simulink model "real_resource_shared_QR_model"  (R2018b)
settings: Solver=FixedStepDiscrete  StartTime=0.0  StopTime=inf  RelTol=1e-3
InitFcn:
  | % Load some variables if running without a test script
  | if ~exist('A','var') || ~exist('B','var') || ~exist('m','var') || ~exist('n','var') || ~exist('p','var') || ~exist('NumberOfCORDICIterations','var')
  |   m = 4; % Number of rows of A and B.
  |   n = 4; % Number of columns of A.
  |   p = 4; % Number of columns of B.
  |   NumberOfCORDICIterations = 52;
  |   A = 2*rand(m,n)-1;
  |   B = 2*rand(m,p)-1;
  | end
libraries: hdlsllib x9, simulink x2
settings Model: DataTypeOverride=Off  Creator=tbryan  LastModifiedBy=tbryan
settings DataIOCC: LimitDataPoints=on  SaveOutput=off  SaveTime=off
settings OptimizationCC: BlockReduction=off  ConditionallyExecuteInputs=off  DefaultParameterBehavior=Inlined  EnhancedBackFolding=on  StrengthReduction=on  PassReuseOutputArgsAs=Individual arguments  OptimizeBlockOrder=speed  DifferentSizesBufferReuse=on
settings DebuggingCC: AlgebraicLoopMsg=error  SingleTaskRateTransMsg=error  IntegerOverflowMsg=none  ParameterDowncastMsg=none  ParameterOverflowMsg=none  ParameterPrecisionLossMsg=none  ParameterTunabilityLossMsg=error  AllowSymbolicDim=off  LibraryContextMissingDiagnostic=none  StrictBusMsg=ErrorOnBusTreatedAsVector  SFUnexpectedBacktrackingDiag=warning  SFNoUnconditionalDefaultTransitionDiag=warning  SFExecutionAtInitializationDiag=none  IntegerSaturationMsg=none
settings HardwareCC: ProdBitPerPointer=32  ProdBitPerSizeT=32  ProdBitPerPtrDiffT=32  ProdLargestAtomicFloat=None  ProdIntDivRoundTo=Undefined  ProdEndianess=Unspecified  ProdWordSize=32  ProdHWDeviceType=ASIC/FPGA->ASIC/FPGA  TargetBitPerLong=64  TargetBitPerPointer=64  TargetBitPerSizeT=64  TargetBitPerPtrDiffT=64  TargetLongLongMode=on  TargetIntDivRoundTo=Zero  TargetEndianess=LittleEndian  TargetWordSize=64  TargetHWDeviceType=Custom Processor->MATLAB Host Computer  ProdEqTarget=off
settings SFSimCC: SimUseLocalCustomCode=off  MATLABDynamicMemAlloc=off
settings RTWCC: SystemTargetFile=ert.tlc  GenCodeOnly=on  TemplateMakefile=ert_default_tmf  GenerateReport=on  RTWUseLocalCustomCode=off  IncludeHyperlinkInReport=on  LaunchReport=on  GenerateTraceInfo=on  GenerateTraceReport=on  GenerateTraceReportSl=on  GenerateTraceReportSf=on  GenerateTraceReportEml=on
settings CodeAppCC: ForceParamTrailComments=on  IgnoreCustomStorageClasses=off  OperatorAnnotations=on  SimulinkDataObjDesc=on  SFDataObjDesc=on  InsertBlockDesc=on
settings ERTTargetCC: GenerateSampleERTMain=on  InlinedParameterPlacement=NonHierarchical  ERTCustomFileTemplate=example_file_process.tlc
settings ConfigComp: CovScope=ReferencedModels  CovMetricSettings=dw  CovHtmlReporting=on  CovSaveCumulativeToWorkspaceVar=on  CovSaveSingleToWorkspaceVar=on  CovExternalEMLEnable=off  CovSFcnEnable=off

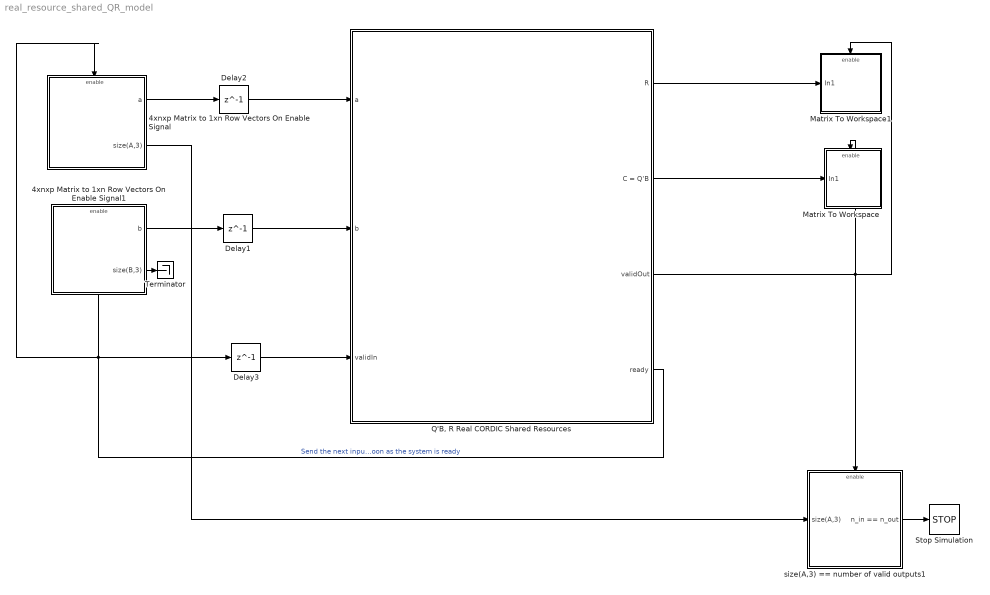
== system real_resource_shared_QR_model ==
  4xnxp Matrix to 1xn Row Vectors On Enable Signal : Subsystem  TreatAsAtomicUnit=on  mask{Matrix=A}
      mask init:
      | obj = get_param(gcbh,'object');
      | constObj = get_param([gcb '/Constant'],'object');
      | constObj.Value = obj.Matrix;
      mask Display: disp(Matrix);
  4xnxp Matrix to 1xn Row Vectors On Enable Signal1 : Subsystem  TreatAsAtomicUnit=on  mask{Matrix=B}
      mask init:
      | obj = get_param(gcbh,'object');
      | constObj = get_param([gcb '/Constant'],'object');
      | constObj.Value = obj.Matrix;
      mask Display: disp(Matrix);
  Delay1 : Delay  DelayLength=1  SampleTime=1
  Delay2 : Delay  DelayLength=1  SampleTime=1
  Delay3 : Delay  DelayLength=1  SampleTime=1
  Matrix To Workspace : Subsystem  mask{VariableName=C}
      mask prompts: VariableName "Variable Name:"
      mask init:
      | obj = get_param(gcbh,'object');
      | twObj = get_param([gcb '/To Workspace'],'object');
      | twObj.VariableName = obj.VariableName;
      mask Display: disp([VariableName,' = Q'' * B']);
  Matrix To Workspace1 : Subsystem  mask{VariableName=R}
      mask prompts: VariableName "Variable Name:"
      mask init:
      | obj = get_param(gcbh,'object');
      | twObj = get_param([gcb '/To Workspace'],'object');
      | twObj.VariableName = obj.VariableName;
      mask Display: disp(VariableName);
  "Q'B, R Real CORDIC Shared Resources" : Subsystem  TreatAsAtomicUnit=on  mask{NumberOfCORDICIterations=NumberOfCORDICIterations, m=m, n=n, p=p}
      mask prompts: NumberOfCORDICIterations "Number of CORDIC Iterations"; m "Number of rows of A and B"; n "Number of columns of A"; p "Number of columns of B"
      mask Display: disp('NumberOfCordicIterations');
  Stop Simulation : Stop
  Terminator : Terminator
  size(A,3) == number of valid outputs1 : Subsystem  TreatAsAtomicUnit=on
  wires:
  4xnxp Matrix to 1xn Row Vectors On Enable Signal/2(size(A,3)) -> size(A,3) == number of valid outputs1/1(size(A,3))
  size(A,3) == number of valid outputs1/1(n_in == n_out) -> Stop Simulation/1
  "Q'B, R Real CORDIC Shared Resources"/2(C = Q'B) -> Matrix To Workspace/1(In1)
  "Q'B, R Real CORDIC Shared Resources"/3(validOut) -> Matrix To Workspace1/Enable, Matrix To Workspace/Enable, size(A,3) == number of valid outputs1/Enable
  4xnxp Matrix to 1xn Row Vectors On Enable Signal/1(a) -> Delay2/1
  4xnxp Matrix to 1xn Row Vectors On Enable Signal1/1(b) -> Delay1/1
  Delay1/1 -> "Q'B, R Real CORDIC Shared Resources"/2(b)
  Delay2/1 -> "Q'B, R Real CORDIC Shared Resources"/1(a)
  Delay3/1 -> "Q'B, R Real CORDIC Shared Resources"/3(validIn)
  "Q'B, R Real CORDIC Shared Resources"/1(R) -> Matrix To Workspace1/1(In1)
  4xnxp Matrix to 1xn Row Vectors On Enable Signal1/2(size(B,3)) -> Terminator/1
  "Q'B, R Real CORDIC Shared Resources"/4(ready) -> 4xnxp Matrix to 1xn Row Vectors On Enable Signal/Enable, 4xnxp Matrix to 1xn Row Vectors On Enable Signal1/Enable, Delay3/1  "Send the next input in as soon as the system is ready"

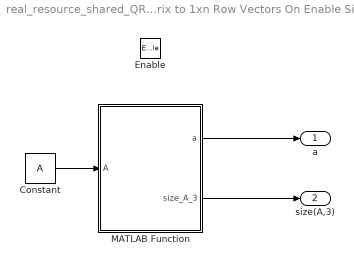
== system real_resource_shared_QR_model/4xnxp Matrix to 1xn Row Vectors On Enable Signal ==
  Enable : EnablePort
  Constant : Constant  Value=A
  MATLAB Function : MATLAB Function  TreatAsAtomicUnit=on
  a : Outport
  size(A,3) : Outport  Port=2
  wires:
  MATLAB Function/1(a) -> a/1
  Constant/1 -> MATLAB Function/1(A)
  MATLAB Function/2(size_A_3) -> size(A,3)/1

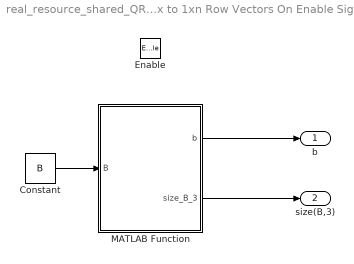
== system real_resource_shared_QR_model/4xnxp Matrix to 1xn Row Vectors On Enable Signal1 ==
  Enable : EnablePort
  Constant : Constant  Value=B
  MATLAB Function : MATLAB Function  TreatAsAtomicUnit=on
  b : Outport
  size(B,3) : Outport  Port=2
  wires:
  MATLAB Function/1(b) -> b/1
  Constant/1 -> MATLAB Function/1(B)
  MATLAB Function/2(size_B_3) -> size(B,3)/1

== system real_resource_shared_QR_model/Matrix To Workspace ==
  In1 : Inport
  Enable : EnablePort
  To Workspace : ToWorkspace  VariableName=C  SampleTime=-1
  wires:
  In1/1 -> To Workspace/1

== system real_resource_shared_QR_model/Matrix To Workspace1 ==
  In1 : Inport
  Enable : EnablePort
  To Workspace : ToWorkspace  VariableName=R  SampleTime=-1
  wires:
  In1/1 -> To Workspace/1

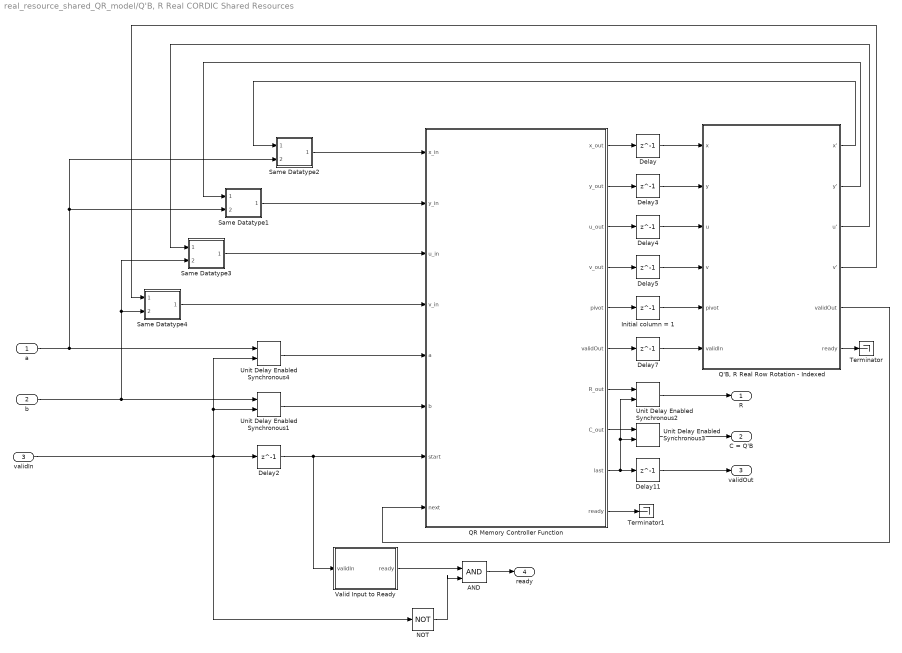
== system real_resource_shared_QR_model/Q'B, R Real CORDIC Shared Resources ==
  a : Inport
  b : Inport  Port=2
  validIn : Inport  Port=3
  AND : Logic  IconShape=distinctive  AllPortsSameDT=off  OutDataTypeStr=boolean
  Delay{,2..5} (5 alike) : Delay  DelayLength=1
  Delay11 : Delay  DelayLength=1  InitialCondition=0
  Delay7 : Delay  DelayLength=1  InitialCondition=0
  Initial column = 1 : Delay  DelayLength=1  InitialCondition=1
  NOT : Logic  Operator=NOT  IconShape=distinctive  AllPortsSameDT=off  OutDataTypeStr=boolean
  "Q'B, R Real Row Rotation - Indexed" : Subsystem  TreatAsAtomicUnit=on  mask{NumberOfCORDICIterations=NumberOfCORDICIterations}
      mask prompts: NumberOfCORDICIterations "Number of CORDIC Iterations"
  QR Memory Controller Function : MATLAB Function  TreatAsAtomicUnit=on
  Same Datatype1 : Subsystem  TreatAsAtomicUnit=on
  Same Datatype2 : Subsystem  TreatAsAtomicUnit=on
  Same Datatype3 : Subsystem  TreatAsAtomicUnit=on
  Same Datatype4 : Subsystem  TreatAsAtomicUnit=on
  Terminator : Terminator
  Terminator1 : Terminator
  Unit Delay Enabled Synchronous{1..4} (4 alike) : hdlsllib/Discrete/Unit Delay Enabled Synchronous  InitialCondition=0.0  SampleTime=-1
      settings: SourceProductName=HDL Coder  SourceProductBaseCode=HD
  Valid Input to Ready : Subsystem  TreatAsAtomicUnit=on  mask{NumberOfCORDICIterations=NumberOfCORDICIterations, m=m, n=n}
      mask prompts: NumberOfCORDICIterations "Number of CORDIC Iterations"; m "Number of rows of A"; n "Number of columns of A"
  R : Outport
  C = Q'B : Outport  Port=2
  validOut : Outport  Port=3
  ready : Outport  Port=4
  wires:
  a/1 -> Unit Delay Enabled Synchronous4/1, Same Datatype2/2(Reference), Same Datatype1/2(Reference)
  b/1 -> Unit Delay Enabled Synchronous1/1, Same Datatype3/2(Reference), Same Datatype4/2(Reference)
  Delay2/1 -> Valid Input to Ready/1(validIn), QR Memory Controller Function/7(start)
  "Q'B, R Real Row Rotation - Indexed"/1(x') -> Same Datatype2/1(Data)
  "Q'B, R Real Row Rotation - Indexed"/2(y') -> Same Datatype1/1(Data)
  "Q'B, R Real Row Rotation - Indexed"/3(u') -> Same Datatype3/1(Data)
  "Q'B, R Real Row Rotation - Indexed"/4(v') -> Same Datatype4/1(Data)
  validIn/1 -> NOT/1, Unit Delay Enabled Synchronous1/2, Unit Delay Enabled Synchronous4/2, Delay2/1
  Same Datatype2/1(DataOut) -> QR Memory Controller Function/1(x_in)
  Same Datatype1/1(DataOut) -> QR Memory Controller Function/2(y_in)
  Same Datatype3/1(DataOut) -> QR Memory Controller Function/3(u_in)
  Same Datatype4/1(DataOut) -> QR Memory Controller Function/4(v_in)
  Unit Delay Enabled Synchronous4/1 -> QR Memory Controller Function/5(a)
  "Q'B, R Real Row Rotation - Indexed"/6(ready) -> Terminator/1
  "Q'B, R Real Row Rotation - Indexed"/5(validOut) -> QR Memory Controller Function/8(next)
  QR Memory Controller Function/1(x_out) -> Delay/1
  QR Memory Controller Function/2(y_out) -> Delay3/1
  QR Memory Controller Function/3(u_out) -> Delay4/1
  QR Memory Controller Function/4(v_out) -> Delay5/1
  QR Memory Controller Function/5(pivot) -> Initial column = 1/1
  QR Memory Controller Function/6(validOut) -> Delay7/1
  Delay/1 -> "Q'B, R Real Row Rotation - Indexed"/1(x)
  Delay3/1 -> "Q'B, R Real Row Rotation - Indexed"/2(y)
  Delay4/1 -> "Q'B, R Real Row Rotation - Indexed"/3(u)
  Delay5/1 -> "Q'B, R Real Row Rotation - Indexed"/4(v)
  Initial column = 1/1 -> "Q'B, R Real Row Rotation - Indexed"/5(pivot)
  Delay7/1 -> "Q'B, R Real Row Rotation - Indexed"/6(validIn)
  QR Memory Controller Function/7(R_out) -> Unit Delay Enabled Synchronous2/1
  QR Memory Controller Function/8(C_out) -> Unit Delay Enabled Synchronous3/1
  QR Memory Controller Function/9(last) -> Unit Delay Enabled Synchronous3/2, Unit Delay Enabled Synchronous2/2, Delay11/1
  Delay11/1 -> validOut/1
  Unit Delay Enabled Synchronous1/1 -> QR Memory Controller Function/6(b)
  Unit Delay Enabled Synchronous2/1 -> R/1
  Unit Delay Enabled Synchronous3/1 -> C = Q'B/1
  QR Memory Controller Function/10(ready) -> Terminator1/1
  AND/1 -> ready/1
  Valid Input to Ready/1(ready) -> AND/1
  NOT/1 -> AND/2

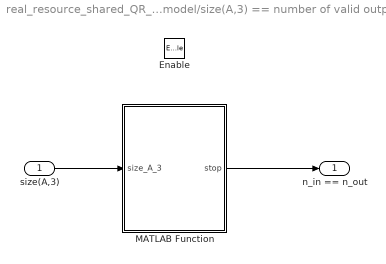
== system real_resource_shared_QR_model/size(A,3) == number of valid outputs1 ==
  size(A,3) : Inport
  Enable : EnablePort
  MATLAB Function : MATLAB Function  TreatAsAtomicUnit=on
  n_in == n_out : Outport
  wires:
  MATLAB Function/1(stop) -> n_in == n_out/1
  size(A,3)/1 -> MATLAB Function/1(size_A_3)

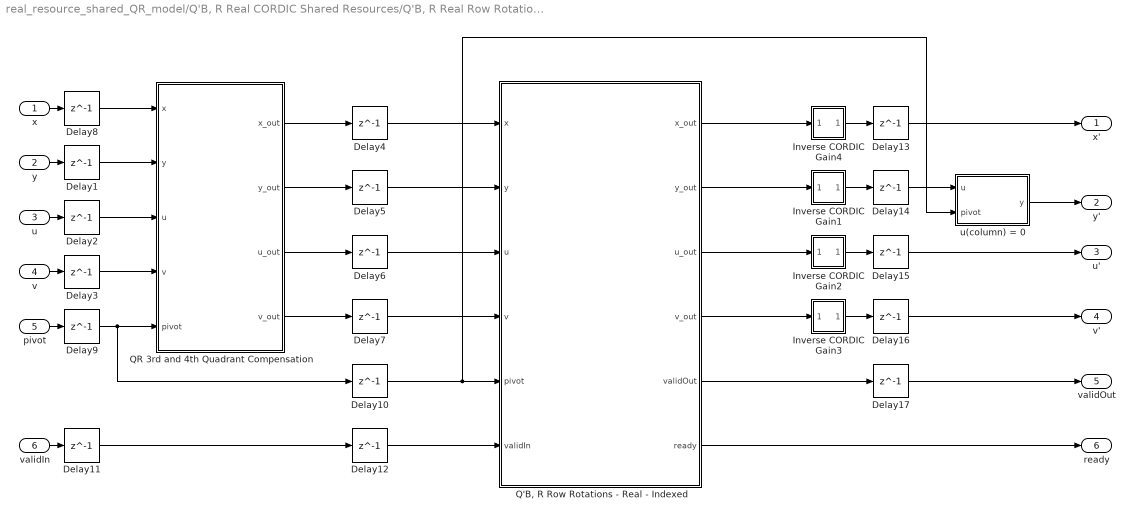
== system real_resource_shared_QR_model/Q'B, R Real CORDIC Shared Resources/Q'B, R Real Row Rotation - Indexed ==
  x : Inport
  y : Inport  Port=2
  u : Inport  Port=3
  v : Inport  Port=4
  pivot : Inport  Port=5
  validIn : Inport  Port=6
  Delay{1..8,11..17} (15 alike) : Delay  DelayLength=1
  Delay10 : Delay  DelayLength=1  InitialCondition=1
  Delay9 : Delay  DelayLength=1  InitialCondition=1
  Inverse CORDIC Gain1 : Subsystem  TreatAsAtomicUnit=on  mask{NumberOfCORDICIterations=NumberOfCORDICIterations}
      mask prompts: NumberOfCORDICIterations "Number of CORDIC Iterations"
      mask Display: disp('1/An')
  Inverse CORDIC Gain2 : Subsystem  TreatAsAtomicUnit=on  mask{NumberOfCORDICIterations=NumberOfCORDICIterations}
      mask prompts: NumberOfCORDICIterations "Number of CORDIC Iterations"
      mask Display: disp('1/An')
  Inverse CORDIC Gain3 : Subsystem  TreatAsAtomicUnit=on  mask{NumberOfCORDICIterations=NumberOfCORDICIterations}
      mask prompts: NumberOfCORDICIterations "Number of CORDIC Iterations"
      mask Display: disp('1/An')
  Inverse CORDIC Gain4 : Subsystem  TreatAsAtomicUnit=on  mask{NumberOfCORDICIterations=NumberOfCORDICIterations}
      mask prompts: NumberOfCORDICIterations "Number of CORDIC Iterations"
      mask Display: disp('1/An')
  "Q'B, R Row Rotations - Real - Indexed" : Subsystem  TreatAsAtomicUnit=on  mask{NumberOfCORDICIterations=NumberOfCORDICIterations}
      mask prompts: NumberOfCORDICIterations "Number of CORDIC Iterations"
  QR 3rd and 4th Quadrant Compensation : MATLAB Function  TreatAsAtomicUnit=on
  u(column) = 0 : MATLAB Function  TreatAsAtomicUnit=on
  x' : Outport
  y' : Outport  Port=2
  u' : Outport  Port=3
  v' : Outport  Port=4
  validOut : Outport  Port=5
  ready : Outport  Port=6
  wires:
  u(column) = 0/1(y) -> y'/1
  Delay9/1 -> Delay10/1, QR 3rd and 4th Quadrant Compensation/5(pivot)
  pivot/1 -> Delay9/1
  Delay10/1 -> u(column) = 0/2(pivot), "Q'B, R Row Rotations - Real - Indexed"/5(pivot)
  Delay12/1 -> "Q'B, R Row Rotations - Real - Indexed"/6(validIn)
  Delay3/1 -> QR 3rd and 4th Quadrant Compensation/4(v)
  Delay1/1 -> QR 3rd and 4th Quadrant Compensation/2(y)
  y/1 -> Delay1/1
  Delay2/1 -> QR 3rd and 4th Quadrant Compensation/3(u)
  Delay8/1 -> QR 3rd and 4th Quadrant Compensation/1(x)
  "Q'B, R Row Rotations - Real - Indexed"/6(ready) -> ready/1
  Delay17/1 -> validOut/1
  "Q'B, R Row Rotations - Real - Indexed"/5(validOut) -> Delay17/1
  Delay16/1 -> v'/1
  Delay15/1 -> u'/1
  Delay13/1 -> x'/1
  Delay11/1 -> Delay12/1
  validIn/1 -> Delay11/1
  "Q'B, R Row Rotations - Real - Indexed"/2(y_out) -> Inverse CORDIC Gain1/1(In1)
  Delay14/1 -> u(column) = 0/1(u)
  Inverse CORDIC Gain1/1(Out1) -> Delay14/1
  "Q'B, R Row Rotations - Real - Indexed"/4(v_out) -> Inverse CORDIC Gain3/1(In1)
  "Q'B, R Row Rotations - Real - Indexed"/3(u_out) -> Inverse CORDIC Gain2/1(In1)
  "Q'B, R Row Rotations - Real - Indexed"/1(x_out) -> Inverse CORDIC Gain4/1(In1)
  Delay7/1 -> "Q'B, R Row Rotations - Real - Indexed"/4(v)
  Delay6/1 -> "Q'B, R Row Rotations - Real - Indexed"/3(u)
  Delay5/1 -> "Q'B, R Row Rotations - Real - Indexed"/2(y)
  Delay4/1 -> "Q'B, R Row Rotations - Real - Indexed"/1(x)
  Inverse CORDIC Gain2/1(Out1) -> Delay15/1
  v/1 -> Delay3/1
  u/1 -> Delay2/1
  x/1 -> Delay8/1
  Inverse CORDIC Gain4/1(Out1) -> Delay13/1
  Inverse CORDIC Gain3/1(Out1) -> Delay16/1
  QR 3rd and 4th Quadrant Compensation/4(v_out) -> Delay7/1
  QR 3rd and 4th Quadrant Compensation/2(y_out) -> Delay5/1
  QR 3rd and 4th Quadrant Compensation/3(u_out) -> Delay6/1
  QR 3rd and 4th Quadrant Compensation/1(x_out) -> Delay4/1

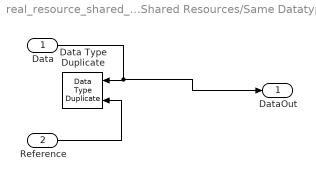
== system real_resource_shared_QR_model/Q'B, R Real CORDIC Shared Resources/Same Datatype1 ==
  Data : Inport
  Reference : Inport  Port=2
  Data Type Duplicate : DataTypeDuplicate
  DataOut : Outport
  wires:
  Data/1 -> Data Type Duplicate/1, DataOut/1
  Reference/1 -> Data Type Duplicate/2

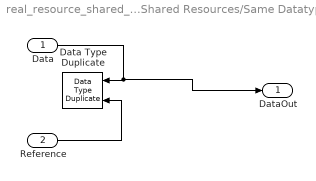
== system real_resource_shared_QR_model/Q'B, R Real CORDIC Shared Resources/Same Datatype2 ==
  Data : Inport
  Reference : Inport  Port=2
  Data Type Duplicate : DataTypeDuplicate
  DataOut : Outport
  wires:
  Data/1 -> Data Type Duplicate/1, DataOut/1
  Reference/1 -> Data Type Duplicate/2

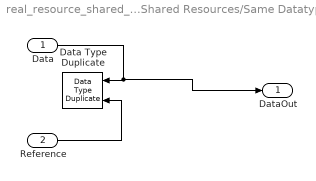
== system real_resource_shared_QR_model/Q'B, R Real CORDIC Shared Resources/Same Datatype3 ==
  Data : Inport
  Reference : Inport  Port=2
  Data Type Duplicate : DataTypeDuplicate
  DataOut : Outport
  wires:
  Data/1 -> Data Type Duplicate/1, DataOut/1
  Reference/1 -> Data Type Duplicate/2

== system real_resource_shared_QR_model/Q'B, R Real CORDIC Shared Resources/Same Datatype4 ==
  Data : Inport
  Reference : Inport  Port=2
  Data Type Duplicate : DataTypeDuplicate
  DataOut : Outport
  wires:
  Data/1 -> Data Type Duplicate/1, DataOut/1
  Reference/1 -> Data Type Duplicate/2

== system real_resource_shared_QR_model/Q'B, R Real CORDIC Shared Resources/Valid Input to Ready ==
  validIn : Inport
  MATLAB Function : MATLAB Function  TreatAsAtomicUnit=on
  ready : Outport
  wires:
  validIn/1 -> MATLAB Function/1(validIn)
  MATLAB Function/1(ready) -> ready/1

== system real_resource_shared_QR_model/Q'B, R Real CORDIC Shared Resources/Q'B, R Real Row Rotation - Indexed/Inverse CORDIC Gain1 ==
  In1 : Inport
  Inverse CORDIC Gain : Gain  Gain=1/prod(sqrt(1+2.^(-2*(0:double(NumberOfCORDICIterations)-1))))  OutDataTypeStr=Inherit: Same as input
  Out1 : Outport
  wires:
  Inverse CORDIC Gain/1 -> Out1/1
  In1/1 -> Inverse CORDIC Gain/1

== system real_resource_shared_QR_model/Q'B, R Real CORDIC Shared Resources/Q'B, R Real Row Rotation - Indexed/Inverse CORDIC Gain2 ==
  In1 : Inport
  Inverse CORDIC Gain : Gain  Gain=1/prod(sqrt(1+2.^(-2*(0:double(NumberOfCORDICIterations)-1))))  OutDataTypeStr=Inherit: Same as input
  Out1 : Outport
  wires:
  Inverse CORDIC Gain/1 -> Out1/1
  In1/1 -> Inverse CORDIC Gain/1

== system real_resource_shared_QR_model/Q'B, R Real CORDIC Shared Resources/Q'B, R Real Row Rotation - Indexed/Inverse CORDIC Gain3 ==
  In1 : Inport
  Inverse CORDIC Gain : Gain  Gain=1/prod(sqrt(1+2.^(-2*(0:double(NumberOfCORDICIterations)-1))))  OutDataTypeStr=Inherit: Same as input
  Out1 : Outport
  wires:
  Inverse CORDIC Gain/1 -> Out1/1
  In1/1 -> Inverse CORDIC Gain/1

== system real_resource_shared_QR_model/Q'B, R Real CORDIC Shared Resources/Q'B, R Real Row Rotation - Indexed/Inverse CORDIC Gain4 ==
  In1 : Inport
  Inverse CORDIC Gain : Gain  Gain=1/prod(sqrt(1+2.^(-2*(0:double(NumberOfCORDICIterations)-1))))  OutDataTypeStr=Inherit: Same as input
  Out1 : Outport
  wires:
  Inverse CORDIC Gain/1 -> Out1/1
  In1/1 -> Inverse CORDIC Gain/1

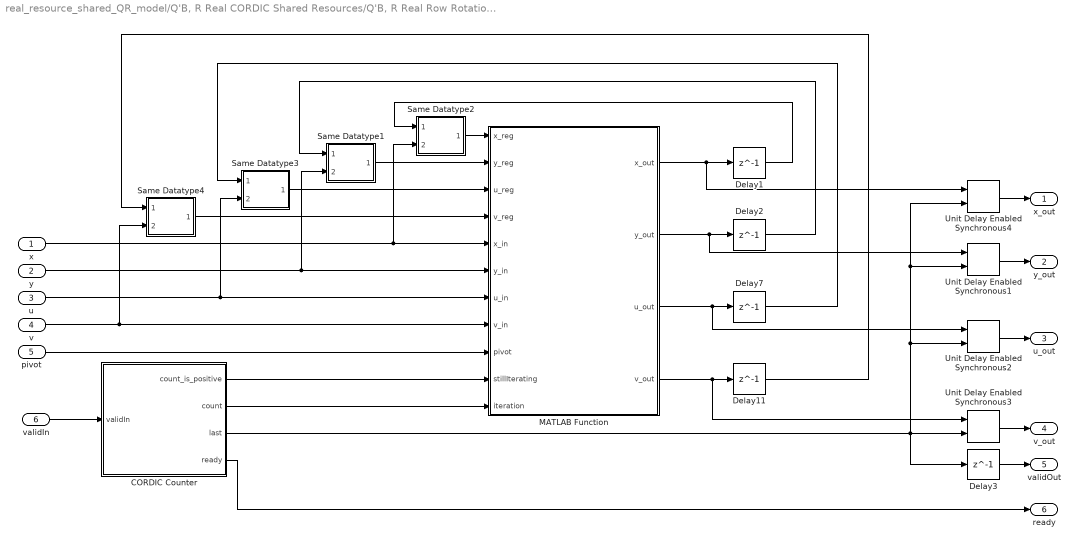
== system real_resource_shared_QR_model/Q'B, R Real CORDIC Shared Resources/Q'B, R Real Row Rotation - Indexed/Q'B, R Row Rotations - Real - Indexed ==
  x : Inport
  y : Inport  Port=2
  u : Inport  Port=3
  v : Inport  Port=4
  pivot : Inport  Port=5
  validIn : Inport  Port=6
  CORDIC Counter : Subsystem  mask{NumberOfCORDICIterations=NumberOfCORDICIterations}
      mask prompts: NumberOfCORDICIterations "Number of CORDIC Iterations"
  Delay{1..3,7,11} (5 alike) : Delay  DelayLength=1
  MATLAB Function : MATLAB Function  TreatAsAtomicUnit=on
  Same Datatype1 : Subsystem  TreatAsAtomicUnit=on
  Same Datatype2 : Subsystem  TreatAsAtomicUnit=on
  Same Datatype3 : Subsystem  TreatAsAtomicUnit=on
  Same Datatype4 : Subsystem  TreatAsAtomicUnit=on
  Unit Delay Enabled Synchronous{1..4} (4 alike) : hdlsllib/Discrete/Unit Delay Enabled Synchronous  InitialCondition=0.0  SampleTime=-1
      settings: SourceProductName=HDL Coder  SourceProductBaseCode=HD
  x_out : Outport
  y_out : Outport  Port=2
  u_out : Outport  Port=3
  v_out : Outport  Port=4
  validOut : Outport  Port=5
  ready : Outport  Port=6
  wires:
  pivot/1 -> MATLAB Function/9(pivot)
  Unit Delay Enabled Synchronous4/1 -> x_out/1
  Unit Delay Enabled Synchronous1/1 -> y_out/1
  Unit Delay Enabled Synchronous2/1 -> u_out/1
  Unit Delay Enabled Synchronous3/1 -> v_out/1
  validIn/1 -> CORDIC Counter/1(validIn)
  CORDIC Counter/4(ready) -> ready/1
  CORDIC Counter/3(last) -> Unit Delay Enabled Synchronous2/2, Unit Delay Enabled Synchronous4/2, Unit Delay Enabled Synchronous1/2, Unit Delay Enabled Synchronous3/2, Delay3/1
  Delay3/1 -> validOut/1
  Same Datatype4/1(DataOut) -> MATLAB Function/4(v_reg)
  Same Datatype3/1(DataOut) -> MATLAB Function/3(u_reg)
  Same Datatype1/1(DataOut) -> MATLAB Function/2(y_reg)
  v/1 -> MATLAB Function/8(v_in), Same Datatype4/2(Reference)
  u/1 -> MATLAB Function/7(u_in), Same Datatype3/2(Reference)
  y/1 -> MATLAB Function/6(y_in), Same Datatype1/2(Reference)
  x/1 -> MATLAB Function/5(x_in), Same Datatype2/2(Reference)
  Same Datatype2/1(DataOut) -> MATLAB Function/1(x_reg)
  MATLAB Function/4(v_out) -> Unit Delay Enabled Synchronous3/1, Delay11/1
  MATLAB Function/3(u_out) -> Unit Delay Enabled Synchronous2/1, Delay7/1
  MATLAB Function/2(y_out) -> Unit Delay Enabled Synchronous1/1, Delay2/1
  MATLAB Function/1(x_out) -> Delay1/1, Unit Delay Enabled Synchronous4/1
  CORDIC Counter/2(count) -> MATLAB Function/11(iteration)
  CORDIC Counter/1(count_is_positive) -> MATLAB Function/10(stillIterating)
  Delay11/1 -> Same Datatype4/1(Data)
  Delay7/1 -> Same Datatype3/1(Data)
  Delay2/1 -> Same Datatype1/1(Data)
  Delay1/1 -> Same Datatype2/1(Data)

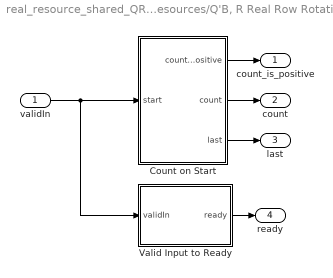
== system real_resource_shared_QR_model/Q'B, R Real CORDIC Shared Resources/Q'B, R Real Row Rotation - Indexed/Q'B, R Row Rotations - Real - Indexed/CORDIC Counter ==
  validIn : Inport
  Count on Start : Subsystem  TreatAsAtomicUnit=on  mask{cmax=NumberOfCORDICIterations - 1}
      mask prompts: cmax "Count Max"
  Valid Input to Ready : Subsystem  TreatAsAtomicUnit=on  mask{NumberOfCORDICIterations=NumberOfCORDICIterations}
      mask prompts: NumberOfCORDICIterations "Number of CORDIC Iterations"
  count_is_positive : Outport
  count : Outport  Port=2
  last : Outport  Port=3
  ready : Outport  Port=4
  wires:
  Valid Input to Ready/1(ready) -> ready/1
  validIn/1 -> Count on Start/1(start), Valid Input to Ready/1(validIn)
  Count on Start/1(count_is_positive) -> count_is_positive/1
  Count on Start/3(last) -> last/1
  Count on Start/2(count) -> count/1

== system real_resource_shared_QR_model/Q'B, R Real CORDIC Shared Resources/Q'B, R Real Row Rotation - Indexed/Q'B, R Row Rotations - Real - Indexed/Same Datatype1 ==
  Data : Inport
  Reference : Inport  Port=2
  Data Type Duplicate : DataTypeDuplicate
  DataOut : Outport
  wires:
  Data/1 -> Data Type Duplicate/1, DataOut/1
  Reference/1 -> Data Type Duplicate/2

== system real_resource_shared_QR_model/Q'B, R Real CORDIC Shared Resources/Q'B, R Real Row Rotation - Indexed/Q'B, R Row Rotations - Real - Indexed/Same Datatype2 ==
  Data : Inport
  Reference : Inport  Port=2
  Data Type Duplicate : DataTypeDuplicate
  DataOut : Outport
  wires:
  Data/1 -> Data Type Duplicate/1, DataOut/1
  Reference/1 -> Data Type Duplicate/2

== system real_resource_shared_QR_model/Q'B, R Real CORDIC Shared Resources/Q'B, R Real Row Rotation - Indexed/Q'B, R Row Rotations - Real - Indexed/Same Datatype3 ==
  Data : Inport
  Reference : Inport  Port=2
  Data Type Duplicate : DataTypeDuplicate
  DataOut : Outport
  wires:
  Data/1 -> Data Type Duplicate/1, DataOut/1
  Reference/1 -> Data Type Duplicate/2

== system real_resource_shared_QR_model/Q'B, R Real CORDIC Shared Resources/Q'B, R Real Row Rotation - Indexed/Q'B, R Row Rotations - Real - Indexed/Same Datatype4 ==
  Data : Inport
  Reference : Inport  Port=2
  Data Type Duplicate : DataTypeDuplicate
  DataOut : Outport
  wires:
  Data/1 -> Data Type Duplicate/1, DataOut/1
  Reference/1 -> Data Type Duplicate/2

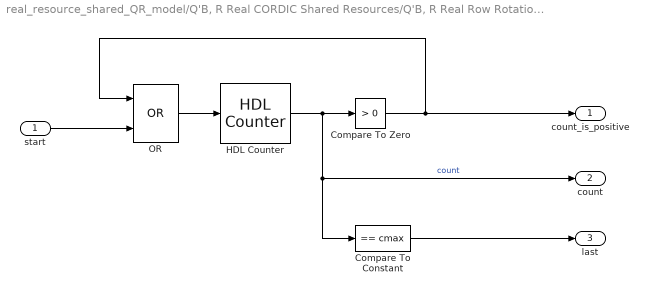
== system real_resource_shared_QR_model/Q'B, R Real CORDIC Shared Resources/Q'B, R Real Row Rotation - Indexed/Q'B, R Row Rotations - Real - Indexed/CORDIC Counter/Count on Start ==
  start : Inport
  Compare To Constant : simulink/Logic and Bit Operations/Compare To Constant  relop===  const=cmax  OutDataTypeStr=boolean
  Compare To Zero : simulink/Logic and Bit Operations/Compare To Zero  relop=>  OutDataTypeStr=boolean
  HDL Counter : hdlsllib/Sources/HDL Counter  CountType=Count limited  CountInit=0  CountStep=1  CountMax=cmax  CountFromType=Initial value  CountFrom=0  CountResetPort=off  CountLoadPort=off  CountEnbPort=on  CountDirPort=off  CountDataType=Unsigned  CountWordLen=nextpow2(cmax+1)  CountFracLen=0  CountSampTime=1
      settings: SourceProductBaseCode=HD
  OR : Logic  Operator=OR  IconShape=distinctive  AllPortsSameDT=off  OutDataTypeStr=boolean
  count_is_positive : Outport
  count : Outport  Port=2
  last : Outport  Port=3
  wires:
  OR/1 -> HDL Counter/1
  Compare To Zero/1 -> OR/1, count_is_positive/1
  start/1 -> OR/2
  HDL Counter/1 -> Compare To Constant/1, count/1, Compare To Zero/1  "count"
  Compare To Constant/1 -> last/1

== system real_resource_shared_QR_model/Q'B, R Real CORDIC Shared Resources/Q'B, R Real Row Rotation - Indexed/Q'B, R Row Rotations - Real - Indexed/CORDIC Counter/Valid Input to Ready ==
  validIn : Inport
  MATLAB Function : MATLAB Function  TreatAsAtomicUnit=on
  ready : Outport
  wires:
  MATLAB Function/1(ready_out) -> ready/1
  validIn/1 -> MATLAB Function/1(validIn)

== matlab function real_resource_shared_QR_model/4xnxp Matrix to 1xn Row Vectors On Enable Signal1/MATLAB Function ==
  settings: fimath=fimath('RoundingMethod','Floor','OverflowAction','Wrap')
  data: b output; B input; size_B_3 output
function [b,size_B_3] = matrix_to_row_vectors_4x4(B)
    persistent p
    if isempty(p)
        p = 1;
    end
    b = reshape(B(:,:,p),1,size(B,1)*size(B,2));
    p = p + 1;
    if p>size(B,3)
        p = 1;
    end
    size_B_3 = size(B,3);
end

== matlab function real_resource_shared_QR_model/Q'B, R Real CORDIC Shared Resources/Q'B, R Real Row Rotation - Indexed/Q'B, R Row Rotations - Real - Indexed/MATLAB Function ==
  settings: fimath=fimath('RoundingMethod','Floor','OverflowAction','Wrap')
  data: x_reg input; y_reg input; u_reg input; v_reg input; x_in input; y_in input; u_in input; x_out output; y_out output; u_out output; v_in input; pivot input size=1; stillIterating input; iteration input size=1; v_out output
function [x_out,y_out,u_out,v_out] = cordic_qr_row_rotation(...
        x_reg,y_reg,u_reg,v_reg,...
        x_in,y_in,u_in,v_in,...
        pivot,...
        stillIterating, iteration)
    % This is one CORDIC rotation for the QR decomposition.
    % In the matrix equation A*X = B
    % x and y form R from A
    % u and v form Q'*B from B
    
    % Initialize output variables
    x_out = x_in;
    y_out = y_in;
    u_out = u_in;
    v_out = v_in;
    
    if pivot <= length(y_in)
        if stillIterating
            % The next values are the previous values from the register
            x = x_reg;
            y = y_reg;
            u = u_reg;
            v = v_reg;
        else
            % The next values are the new input values
            x = x_in;
            y = y_in;
            u = u_in;
            v = v_in;
        end
        
        % Right shift the inputs for CORDIC rotations.
        x1 = bitsra(x, iteration);
        y1 = bitsra(y, iteration);
        u1 = bitsra(u, iteration);
        v1 = bitsra(v, iteration);
        if real(y(pivot)) < 0
            % Counter-clockwise rotation
            x_out(:) = x - y1;
            y_out(:) = y + x1;
            
            u_out(:) = u - v1;
            v_out(:) = v + u1;
        else
            % Clockwise rotation
            x_out(:) = x + y1;
            y_out(:) = y - x1;
            
            u_out(:) = u + v1;
            v_out(:) = v - u1;
        end
    end
end

== matlab function real_resource_shared_QR_model/Q'B, R Real CORDIC Shared Resources/Valid Input to Ready/MATLAB Function ==
  settings: fimath=fimath('RoundingMethod','Floor','OverflowAction','Wrap')
  data: validIn input boolean size=1; ready output boolean size=1; NumberOfCORDICIterations parameter size=1; m parameter size=1; n parameter size=1
function ready = valid_in_ready_out(validIn, NumberOfCORDICIterations,m, n)
    persistent count
    if isempty(count)
        count = uint32(0);
    end
    % Constants
    if m<n
        number_of_lower_triangular_entries = m*(m-1)/2;
    else
        number_of_lower_triangular_entries = n*(n-1)/2 + (m-n)*n;
    end
    count_to_ready = (number_of_lower_triangular_entries+5) * NumberOfCORDICIterations;
    if validIn
        count(:) = 1;
        ready = false;
    elseif count > count_to_ready
        ready = true;
        count(:) = 0;
    elseif count > 0
        count(:) = count + 1;
        ready = false;
    else
        ready = true;
    end
end

== matlab function real_resource_shared_QR_model/Q'B, R Real CORDIC Shared Resources/QR Memory Controller Function ==
  data: x_in input size=[1,n]; y_in input size=[1,n]; u_in input size=[1,p]; v_in input size=[1,p]; a input size=[1,m*n]; x_out output size=[1,n]; b input size=[1,m*p]; start input boolean size=1; next input boolean size=1; y_out output size=[1,n]; u_out output size=[1,p]; v_out output size=[1,p]; pivot output size=1; validOut output; R_out output size=[m,n]; C_out output size=[m,p]; last output boolean size=1; m parameter size=1; n parameter size=1; p parameter size=1; ready output boolean size=1
function [x_out,...
        y_out,...
        u_out,...
        v_out,...
        pivot,...
        validOut,...
        R_out,...
        C_out,...
        last,...
        ready]...
          = qr_memory_controller(...
        x_in,...
        y_in,...
        u_in,...
        v_in,...
        a,...
        b,...
        start,...
        next,...
        m,...
        n,...
        p)
    
    persistent R C i pPivot count pReady
    if isempty(R)
        % Initialize persistent variables
        R = zeros(m,n,'like',a);
        C = zeros(m,p,'like',b);
        pPivot = uint16(1);
        i = uint16(1);
        count = uint16(0);
        pReady = true;
    end
    mn = min(m,n);
    if m<n
        number_of_lower_triangular_entries = m*(m-1)/2;
    else
        number_of_lower_triangular_entries = n*(n-1)/2 + (m-n)*n;
    end
    last = false;
    validOut = false;
    x_out = zeros(1,n,'like',a);
    y_out = zeros(1,n,'like',a);
    u_out = zeros(1,p,'like',b);
    v_out = zeros(1,p,'like',b);
    if start
        count(:) = 1;
        % Start with a new matrix
        % Overwrite A with R
        R(:) = a;
        % Overwrite B with C = Q'B
        C(:) = b;
        % Initial indices
        pPivot(:) = 1;
        i(:) = 2;
        if pPivot<=mn && i<=m
            % Initial rows to operate over
            x_out = R(pPivot,:);
            y_out = R(i,:);
            u_out = C(pPivot,:);
            v_out = C(i,:);
        end
        pReady = false;
        validOut = true;
    elseif next && count ~= 0
        count(:) = count + 1;
        % Update previous pair of rows and get next pair
        if pPivot<=mn && i<=m
            % Update R with previous values
            R(pPivot,:) = x_in;
            R(i,:) = y_in;
            % Update C with previous values
            C(pPivot,:) = u_in;
            C(i,:) = v_in;
            % Increment loop
            i(:) = i + 1;  % Inner loop
            if i > m
                pPivot(:) = pPivot + 1;  % Outer loop
                i(:) = pPivot + 1;
            end
            if pPivot <= mn && i <= m
                % Next rows to operate over
                x_out = R(pPivot,:);
                y_out = R(i,:);
                u_out = C(pPivot,:);
                v_out = C(i,:);
            end
        end
        validOut = true;
    end
    if count > number_of_lower_triangular_entries
        last = true;
        count(:) = 0;
        pReady = true;
    end
    ready = pReady;
    pivot = pPivot;
    R_out = R;
    C_out = C;
    %{
      for j=1:n
        for i=j+1:m
          % Apply Givens rotations, zeroing out the i-jth entry below
          % the diagonal.  Apply the same rotations to the columns of Q
          % that are applied to the rows of R so that Q'*A = R.
          [R(j,:),R(i,:),C(j,:),C(i,:)] = ...
              cordicgivens(R(j,:),R(i,:),C(j,:),C(i,:),j,niter,Kn);
        end
      end
    %}
    
end

== matlab function real_resource_shared_QR_model/Q'B, R Real CORDIC Shared Resources/Q'B, R Real Row Rotation - Indexed/Q'B, R Row Rotations - Real - Indexed/CORDIC Counter/Valid Input to Ready/MATLAB Function ==
  settings: fimath=fimath('RoundingMethod','Floor','OverflowAction','Wrap')
  data: validIn input; ready_out output; NumberOfCORDICIterations parameter size=1
function ready_out = valid_in_ready_out(validIn, NumberOfCORDICIterations)

    persistent count
    if isempty(count)
        count = fi(0,0,nextpow2(NumberOfCORDICIterations+1),0,...
            'OverflowAction','Wrap',...
            'RoundingMethod','Floor',...
            'SumMode','KeepLSB',...
            'SumWordLength',nextpow2(NumberOfCORDICIterations+1));
    end
    if validIn
        count(:) = 0;
        ready_out = false;
    elseif count >= NumberOfCORDICIterations - 1 %3
        ready_out = true;
        count(:) = 0;
    else
        count(:) = count + 1;
        ready_out = false;
    end
end

== matlab function real_resource_shared_QR_model/size(A,3) == number of valid outputs1/MATLAB Function ==
  settings: fimath=fimath('RoundingMethod','Floor','OverflowAction','Wrap')
  data: stop output; size_A_3 input
function stop  = matrix_to_row_vectors_4x4(size_A_3)
    persistent p
    if isempty(p)
        p = 0;
    end
    p = p + 1;
    stop = p >= size_A_3;
end

== matlab function real_resource_shared_QR_model/Q'B, R Real CORDIC Shared Resources/Q'B, R Real Row Rotation - Indexed/QR 3rd and 4th Quadrant Compensation ==
  settings: fimath=fimath('RoundingMethod','Floor','OverflowAction','Wrap')
  data: x input; y input; u input; x_out output; y_out output; u_out output; v input; v_out output; pivot input size=1
function [x_out,y_out,u_out,v_out] = quadrant_compensation(x,y,u,v,pivot)
    
    if pivot <= length(x) && real(x(pivot))<0
        % Compensation for 3rd and 4th quadrants
        x_out = -x;
        y_out = -y;
        
        u_out = -u;
        v_out = -v;
        
    else
        x_out = x;
        y_out = y;
        
        u_out = u;
        v_out = v;
        
    end
end

== matlab function real_resource_shared_QR_model/Q'B, R Real CORDIC Shared Resources/Q'B, R Real Row Rotation - Indexed/u(column) = 0 ==
  settings: fimath=fimath('RoundingMethod','Floor','OverflowAction','Wrap')
  data: u input; y output; pivot input
function y = set_column_equal_to_zero(u,pivot)
    
    y = u;
    if pivot <= length(y)
        y(pivot) = cast(0,'like',u);
    end
    
end

== matlab function real_resource_shared_QR_model/4xnxp Matrix to 1xn Row Vectors On Enable Signal/MATLAB Function ==
  settings: fimath=fimath('RoundingMethod','Floor','OverflowAction','Wrap')
  data: a output; A input; size_A_3 output
function [a,size_A_3] = matrix_to_row_vectors_4x4(A)
    persistent p
    if isempty(p)
        p = 1;
    end
    a = reshape(A(:,:,p),1,size(A,1)*size(A,2));
    p = p + 1;
    if p>size(A,3)
        p = 1;
    end
    size_A_3 = size(A,3);
end
